simulink model "xhand_sphere_tube_r50_v3"  (R2022b)
settings: Solver=VariableStepAuto  StartTime=0.0  StopTime=5  RelTol=1e-3
InitFcn:
  | clc;
  | clear;
  | addpath('H:\研究生\新建文件夹\xhand\meshes');
  | radium=0.055
  | global flag_gravity;
  | flag_gravity=0;
undefined symbols (not defined in the file): X, Y, Z
libraries: sm_lib x125, nesl_utility x27, Contact_Forces_Lib x26
(part 5 of 5)

== matlab function xhand_sphere_tube_r50_v3/contact position tip ==
  data: x input; xx output; y input; q1 input; q2 input; yy output; zz output
function [xx,yy,zz] = fcn(x,y,q1,q2)
theta01=45*3.14/180;    %初始位置和xz平面夹角
theta02=15*3.14/180;    %初始位置和xy平面夹角
trans0=[y*cos(q2+theta01) y*sin(q2+theta01) x 1];
p011=[19.35 -59.86 24.22 1]; p012=[15.18 -55.55 24.40 1];   %大拇指侧摆位置两点
p01=(p011+p012)/2;  p01(4)=1;
direction=[1 -1 0 1];
p021=[26.41 -44.30 24.60 1]; p022=[25.97 -44.85 27.52 1];   %大拇指近指滑轮两点
p02=(p021+p022)/2; p02(4)=1;
a1x=abs(atan(direction(2)/direction(3)));
a1y=abs(atan(direction(1)/(direction(2)^2+direction(3)^2)^0.5));
position01=p02*[[1 0 0 0]' [0 1 0 0]' [0 0 1 0]' [-p01(1) -p01(2) -p01(3) 1]']'...
    *[[1 0 0 0]' [0 cos(a1x) sin(a1x) 0]' [0 -sin(a1x) cos(a1x) 0]' [0 0 0 1]']'*[[cos(a1y) 0 -sin(a1y) 0]' [0 1 0 0]'  [sin(a1y) 0 cos(a1y) 0]' [0 0 0 1]']'...
    *[[cos(theta02) sin(theta02) 0 0]' [-sin(theta02) cos(theta02) 0 0]' [0 0 1 0]' [0 0 0 1]']'...
    *[[cos(-a1y) 0 -sin(-a1y) 0]' [0 1 0 0]'  [sin(-a1y) 0 cos(-a1y) 0]' [0 0 0 1]']'*[[1 0 0 0]' [0 cos(-a1x) sin(-a1x) 0]' [0 -sin(-a1x) cos(-a1x) 0]' [0 0 0 1]']'...
    *[[1 0 0 0]' [0 1 0 0]' [0 0 1 0]' [p01(1) p01(2) p01(3) 1]']';
position02=position01+trans0; position02(4)=1;
position0=position02*[[1 0 0 0]' [0 1 0 0]' [0 0 1 0]' [-p01(1) -p01(2) -p01(3) 1]']'...
    *[[1 0 0 0]' [0 cos(a1x) sin(a1x) 0]' [0 -sin(a1x) cos(a1x) 0]' [0 0 0 1]']'*[[cos(a1y) 0 -sin(a1y) 0]' [0 1 0 0]'  [sin(a1y) 0 cos(a1y) 0]' [0 0 0 1]']'...
    *[[cos(-q1-theta02) sin(-q1-theta02) 0 0]' [-sin(-q1-theta02) cos(-q1-theta02) 0 0]' [0 0 1 0]' [0 0 0 1]']'...
    *[[cos(-a1y) 0 -sin(-a1y) 0]' [0 1 0 0]'  [sin(-a1y) 0 cos(-a1y) 0]' [0 0 0 1]']'*[[1 0 0 0]' [0 cos(-a1x) sin(-a1x) 0]' [0 -sin(-a1x) cos(-a1x) 0]' [0 0 0 1]']'...
    *[[1 0 0 0]' [0 1 0 0]' [0 0 1 0]' [p01(1) p01(2) p01(3) 1]']';
position0=position0(1:3);
p0=position0;
xx=p0(1);
yy=p0(2);
zz=p0(3);

== matlab function xhand_sphere_tube_r50_v3/MATLAB Function7 ==
  data: u input; flag_gravity output; f input
function flag_gravity = fcn(u,f)
if u>0.01
    flag_gravity=1;
else
    flag_gravity=f;
end

== matlab function xhand_sphere_tube_r50_v3/MATLAB Function1 ==
  data: a1 input; j output; a2 input; r1 input; l1 input; r2 input; l2 input
function j = fcn(a1,a2,r1,l1,r2,l2)

j=zeros(6,4);

a_ta=-1.17; %侧摆的角度
theta1=pi/180*15;   %拇指与xoy平面的角度
theta2=pi/180*45;   %拇指与xoz平面的角度
l=36.17*0.001;

 j(1,1)=-l1*cos(theta2)*cos(a_ta+theta1)*sin(a1+r1)-l1*sin(theta2)*cos(a1+r1);
 j(2,1)=-l1*sin(theta2)*cos(a_ta+theta1)*sin(a1+r1)+l1*cos(theta2)*cos(a1+r1);
 j(3,1)=-l1*sin(a_ta+theta1)*sin(a1+r1);

 j(4,3)=-l*cos(theta2)*cos(a_ta+theta1)*sin(a1)-l2*cos(theta2)*cos(a_ta+theta1)*sin(a1+a2+r2)-l*sin(theta2)*cos(a1)-l2*sin(theta2)*cos(a1+a2+r2);
 j(5,3)=-l*sin(theta2)*cos(a_ta+theta1)*sin(a1)-l2*sin(theta2)*cos(a_ta+theta1)*sin(a1+a2+r2)+l*cos(theta2)*cos(a1)+l2*cos(theta2)*cos(a1+a2+r2);
 j(6,3)=-l*sin(a_ta+theta1)*sin(a1)-l2*sin(a_ta+theta1)*sin(a1+a2+r2);
 j(4,4)=-l2*cos(theta2)*cos(a_ta+theta1)*sin(a1+a2+r2)-l2*sin(theta2)*cos(a1+a2+r2);
 j(5,4)=-l2*sin(theta2)*cos(a_ta+theta1)*sin(a1+a2+r2)+l2*cos(theta2)*cos(a1+a2+r2);
 j(6,4)=-l2*sin(a_ta+theta1)*sin(a1+a2+r2);

== matlab function xhand_sphere_tube_r50_v3/MATLAB Function ==
  data: x1 input; l1 output; x2 input; l2 output; l3 output; l4 output
function [l1,l2,l3,l4] = fcn(x1,x2)

N=[[1 0];[1-18/47 18/47];[1-37.7/47 37.7/47];[0 1]];
l=N*[x1;x2];
l1=l(1);
l2=l(2);
l3=l(3);
l4=l(4);

== matlab function xhand_sphere_tube_r50_v3/MATLAB Function3 ==
  data: y input; r output; z input; l output
function [r,l] = fcn(y,z)
r=atan(z/y);
l=norm([y,z]);

== matlab function xhand_sphere_tube_r50_v3/MATLAB Function5 ==
  data: y input; r output; z input; l output
function [r,l] = fcn(y,z)
r=atan(z/y);
l=norm([y,z]);

== matlab function xhand_sphere_tube_r50_v3/contact position mpip ==
  data: x input; xx output; y input; z input; q1 input; q2 input; yy output; zz output; l output
function [xx,yy,zz,l] = fcn(x,y,z,q1,q2)

xx=0+x;
yy=43.37*cos(q1)+y*cos(q1+q2);
zz=43.37*sin(q1)+y*cos(q1+q2);

xx=xx-1.2;
yy=yy+7.5;
zz=zz+8.5;

l=z;

== matlab function xhand_sphere_tube_r50_v3/contact position ipip ==
  data: x input; xx output; y input; z input; q1 input; q2 input; yy output; zz output; l output
function [xx,yy,zz,l] = fcn(x,y,z,q1,q2)

%在食指坐标系下的坐标值
xx1=0+x;
yy1=37.77*cos(q1)+y*cos(q1+q2);
zz=37.77*sin(q1)+y*cos(q1+q2);

%在与中指坐标系的平行系下的坐标值
alpha=atan(yy1/xx1);
l=norm([xx1,yy1]);
xx2=l*cos(alpha-4*pi/180);
yy2=l*sin(alpha-4*pi/180);

%在种植坐标系下的坐标值
xx=xx2+18.4272*cos(4*pi/180)-1.2;
yy=yy2-18.4272*sin(4*pi/180)+7.5;
zz=zz+8.5;

l=z;
